simulink model "simuMotorFeedforward3"  (R2014a)
settings: Solver=ode45  StartTime=0.0  StopTime=3  MaxStep=0.0001  RelTol=1e-3
values from neighbouring files (symbols this model uses):
  contr = param    [parametres.m]
undefined symbols (not defined in the file or in its folder): param
settings Model: Creator=Etienne  LastModifiedBy=Etienne

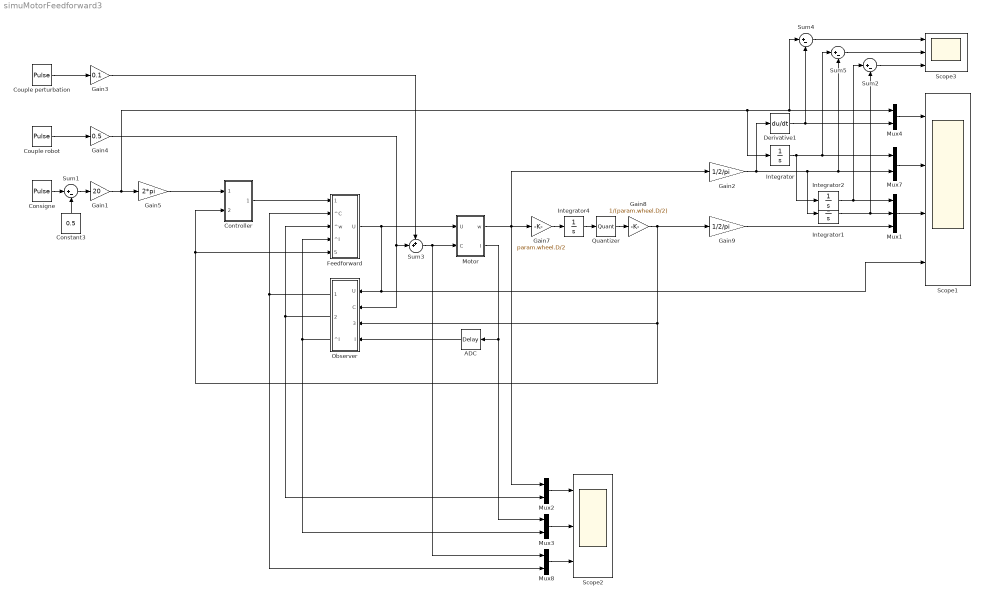
== system simuMotorFeedforward3 ==
  ADC : TransportDelay  DelayTime=param.adc.retard
  Consigne : DiscretePulseGenerator  PulseType=Time based  Period=1  PulseWidth=50  PhaseDelay=0.25/2
  Constant3 : Constant  Value=0.5
  Controller : Subsystem
  Couple perturbation : DiscretePulseGenerator  PulseType=Time based  Period=2/3  PulseWidth=50  PhaseDelay=0.3
  Couple robot : DiscretePulseGenerator  PulseType=Time based  Period=1.5  PulseWidth=50  PhaseDelay=0.1
  Derivative1 : Derivative
  Feedforward : Subsystem
  Gain1 : Gain  Gain=20
  Gain2 : Gain  Gain=1/2/pi
  Gain3 : Gain  Gain=0.1
  Gain4 : Gain  Gain=0.5
  Gain5 : Gain  Gain=2*pi
  Gain7 : Gain  Gain=param.wheel.D/2
  Gain8 : Gain  Gain=1/(param.wheel.D/2)
  Gain9 : Gain  Gain=1/2/pi
  Integrator{,1..2,4} (4 alike) : Integrator
  Motor : Subsystem
  Mux1 : Mux  Inputs=3
  Mux{2..4,7..8} (5 alike) : Mux  Inputs=2
  Observer : Subsystem
  Quantizer : Quantizer  QuantizationInterval=param.codeur.resolution
  Scope1 : Scope  NumInputPorts=4
      settings: TimeRange=3  YMin=-250~-2~-0.5~-30  YMax=200~4~4~30  SaveName=ScopeData2  MaxDataPoints=500000
  Scope2 : Scope  NumInputPorts=3
      settings: TimeRange=3  YMin=-10~-6~-1.5  YMax=25~10~3  MaxDataPoints=500000
  Scope3 : Scope  NumInputPorts=3
      settings: TimeRange=3  YMin=-100~-0.4~-0.005  YMax=150~0.3~0.004000000000000001  SaveName=ScopeData3  MaxDataPoints=500000
  Sum{1..2,4..5} (4 alike) : Sum  Inputs=|+-
  Sum3 : Sum  Inputs=++|
  wires:
  Couple perturbation/1 -> Gain3/1
  Motor/2(I) -> Mux3/1, ADC/1
  Consigne/1 -> Sum1/1
  Sum1/1 -> Gain1/1
  Constant3/1 -> Sum1/2
  Gain2/1 -> Derivative1/1, Integrator1/1, Sum5/2, Mux7/2
  Feedforward/1(U) -> Motor/1(U), Scope1/4, Observer/1(U)
  ADC/1 -> Observer/4(I)
  Mux4/1 -> Scope1/1
  Observer/2(^w) -> Mux2/2, Feedforward/3(^w)
  Observer/3(^I) -> Mux3/2, Feedforward/4(^I)
  Gain1/1 -> Gain5/1, Integrator/1, Mux4/1, Sum4/1
  Gain3/1 -> Sum3/1
  Derivative1/1 -> Mux4/2, Sum4/2
  Mux7/1 -> Scope1/2
  Integrator/1 -> Sum5/1, Mux7/1, Integrator2/1
  Sum4/1 -> Scope3/1
  Sum5/1 -> Scope3/2
  Mux1/1 -> Scope1/3
  Integrator1/1 -> Mux1/2, Sum2/2
  Integrator2/1 -> Mux1/1, Sum2/1
  Sum2/1 -> Scope3/3
  Gain4/1 -> Sum3/2, Observer/2(C)
  Integrator4/1 -> Quantizer/1
  Quantizer/1 -> Gain8/1
  Gain9/1 -> Mux1/3
  Motor/1(w) -> Gain7/1, Gain2/1, Mux2/1
  Gain7/1 -> Integrator4/1
  Mux2/1 -> Scope2/1
  Mux3/1 -> Scope2/2
  Mux8/1 -> Scope2/3
  Gain5/1 -> Controller/1(cons)
  Sum3/1 -> Motor/2(C), Mux8/1
  Couple robot/1 -> Gain4/1
  Controller/1(out) -> Feedforward/1(cons)
  Gain8/1 -> Feedforward/5(teta), Controller/2(teta), Observer/3(teta), Gain9/1
  Observer/1(^C) -> Feedforward/2(^C), Mux8/2

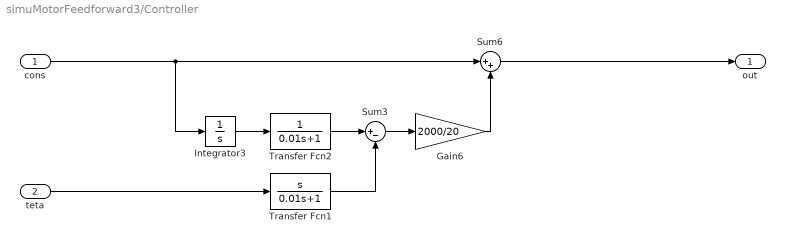
== system simuMotorFeedforward3/Controller ==
  cons : Inport
  teta : Inport  Port=2
  Gain6 : Gain  Gain=2000/20
  Integrator3 : Integrator
  Sum3 : Sum  Inputs=|+-
  Sum6 : Sum  Inputs=|++
  Transfer Fcn1 : TransferFcn  Numerator=[1 0]  Denominator=[0.01 1]
  Transfer Fcn2 : TransferFcn  Denominator=[0.01 1]
  out : Outport
  wires:
  Transfer Fcn2/1 -> Sum3/1
  teta/1 -> Transfer Fcn1/1
  Integrator3/1 -> Transfer Fcn2/1
  cons/1 -> Sum6/1, Integrator3/1
  Sum3/1 -> Gain6/1
  Sum6/1 -> out/1
  Gain6/1 -> Sum6/2
  Transfer Fcn1/1 -> Sum3/2

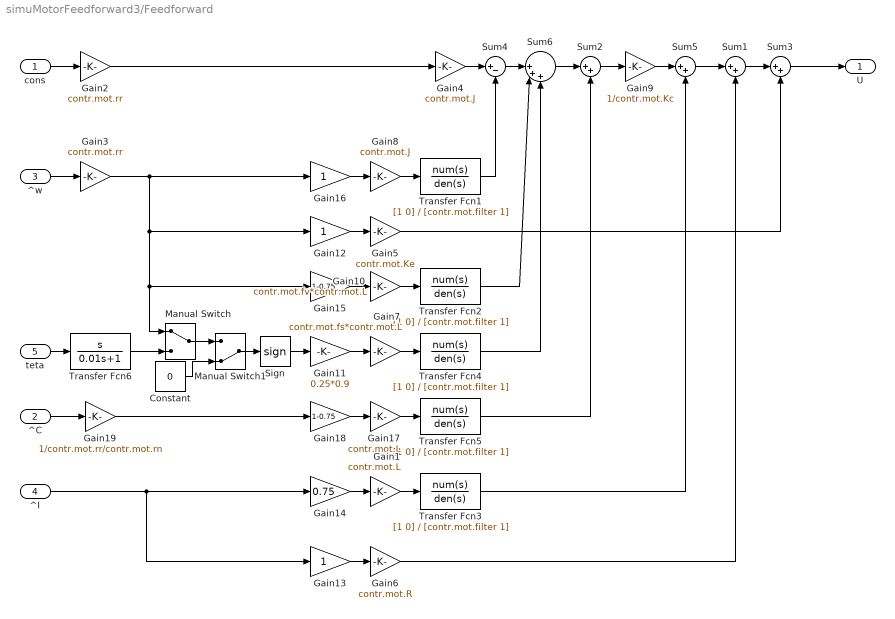
== system simuMotorFeedforward3/Feedforward ==
  cons : Inport
  ^C : Inport  Port=2
  ^w : Inport  Port=3
  ^I : Inport  Port=4
  teta : Inport  Port=5
  Constant : Constant  Value=0
  Gain1 : Gain  Gain=contr.mot.L
  Gain10 : Gain  Gain=contr.mot.fv*contr.mot.L
  Gain11 : Gain  Gain=0.25*0.9
  Gain12 : Gain
  Gain13 : Gain
  Gain14 : Gain  Gain=0.75
  Gain15 : Gain  Gain=1-0.75
  Gain16 : Gain
  Gain17 : Gain  Gain=contr.mot.L
  Gain18 : Gain  Gain=1-0.75
  Gain19 : Gain  Gain=1/contr.mot.rr/contr.mot.rn
  Gain2 : Gain  Gain=contr.mot.rr
  Gain3 : Gain  Gain=contr.mot.rr
  Gain4 : Gain  Gain=contr.mot.J
  Gain5 : Gain  Gain=contr.mot.Ke
  Gain6 : Gain  Gain=contr.mot.R
  Gain7 : Gain  Gain=contr.mot.fs*contr.mot.L
  Gain8 : Gain  Gain=contr.mot.J
  Gain9 : Gain  Gain=1/contr.mot.Kc
  Manual Switch : ManualSwitch
  Manual Switch1 : ManualSwitch  CurrentSetting=0
  Sign : Signum  ZeroCross=off
  Sum{1..3,5} (4 alike) : Sum  Inputs=|++
  Sum4 : Sum  Inputs=|+-
  Sum6 : Sum  Inputs=||+++
  Transfer Fcn{1..5} (5 alike) : TransferFcn  Numerator=[1 0]  Denominator=[contr.mot.filter 1]
  Transfer Fcn6 : TransferFcn  Numerator=[1 0]  Denominator=[0.01 1]
  U : Outport
  wires:
  Gain5/1 -> Sum3/2
  Gain8/1 -> Transfer Fcn1/1
  Gain2/1 -> Gain4/1
  Sum1/1 -> Sum3/1
  Gain6/1 -> Sum1/2
  Sum3/1 -> U/1
  Transfer Fcn1/1 -> Sum4/2
  Transfer Fcn3/1 -> Sum5/2
  Sum5/1 -> Sum1/1
  Gain12/1 -> Gain5/1
  Gain9/1 -> Sum5/1
  Gain1/1 -> Transfer Fcn3/1
  Gain15/1 -> Gain10/1
  Gain16/1 -> Gain8/1
  Gain13/1 -> Gain6/1
  Gain14/1 -> Gain1/1
  Sum4/1 -> Sum6/1
  cons/1 -> Gain2/1
  ^w/1 -> Gain3/1
  ^I/1 -> Gain14/1, Gain13/1
  Gain4/1 -> Sum4/1
  Gain10/1 -> Transfer Fcn2/1
  Transfer Fcn2/1 -> Sum6/2
  Gain7/1 -> Transfer Fcn4/1
  Gain11/1 -> Gain7/1
  Sign/1 -> Gain11/1
  Transfer Fcn4/1 -> Sum6/3
  Gain17/1 -> Transfer Fcn5/1
  Gain18/1 -> Gain17/1
  Sum6/1 -> Sum2/1
  Sum2/1 -> Gain9/1
  Transfer Fcn5/1 -> Sum2/2
  ^C/1 -> Gain19/1
  teta/1 -> Transfer Fcn6/1
  Gain19/1 -> Gain18/1
  Gain3/1 -> Gain16/1, Gain12/1, Gain15/1, Manual Switch/1
  Manual Switch/1 -> Manual Switch1/1
  Transfer Fcn6/1 -> Manual Switch/2
  Constant/1 -> Manual Switch1/2
  Manual Switch1/1 -> Sign/1

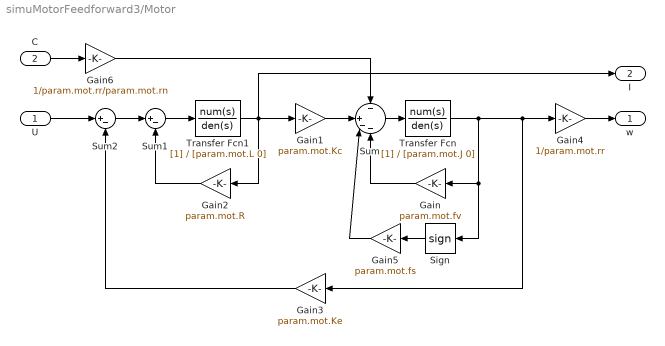
== system simuMotorFeedforward3/Motor ==
  U : Inport
  C : Inport  Port=2
  Gain : Gain  Gain=param.mot.fv
  Gain1 : Gain  Gain=param.mot.Kc
  Gain2 : Gain  Gain=param.mot.R
  Gain3 : Gain  Gain=param.mot.Ke
  Gain4 : Gain  Gain=1/param.mot.rr
  Gain5 : Gain  Gain=param.mot.fs
  Gain6 : Gain  Gain=1/param.mot.rr/param.mot.rn
  Sign : Signum  ZeroCross=off
  Sum : Sum  Inputs=-|+--
  Sum1 : Sum  Inputs=|+-
  Sum2 : Sum  Inputs=|+-
  Transfer Fcn : TransferFcn  Denominator=[param.mot.J 0]
  Transfer Fcn1 : TransferFcn  Denominator=[param.mot.L 0]
  w : Outport
  I : Outport  Port=2
  wires:
  Gain1/1 -> Sum/2
  Transfer Fcn/1 -> Gain3/1, Gain4/1, Sign/1, Gain/1
  Gain3/1 -> Sum2/2
  Sum2/1 -> Sum1/1
  Gain2/1 -> Sum1/2
  Sum1/1 -> Transfer Fcn1/1
  U/1 -> Sum2/1
  C/1 -> Gain6/1
  Gain6/1 -> Sum/1
  Gain4/1 -> w/1
  Sum/1 -> Transfer Fcn/1
  Transfer Fcn1/1 -> Gain1/1, I/1, Gain2/1
  Sign/1 -> Gain5/1
  Gain/1 -> Sum/4
  Gain5/1 -> Sum/3

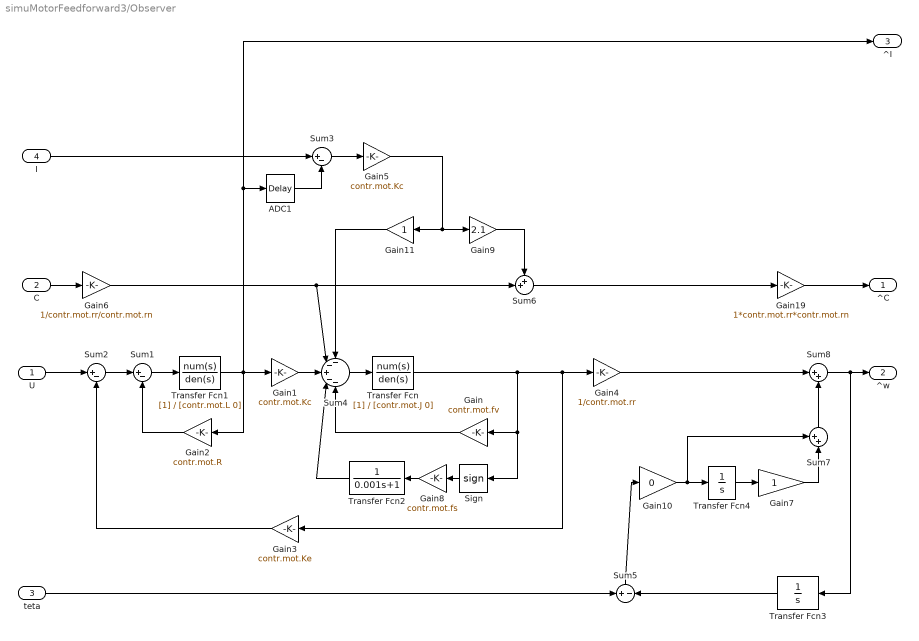
== system simuMotorFeedforward3/Observer ==
  U : Inport
  C : Inport  Port=2
  teta : Inport  Port=3
  I : Inport  Port=4
  ADC1 : TransportDelay  DelayTime=contr.adc.retard
  Gain : Gain  Gain=contr.mot.fv
  Gain1 : Gain  Gain=contr.mot.Kc
  Gain10 : Gain  Gain=0
  Gain11 : Gain
  Gain19 : Gain  Gain=1*contr.mot.rr*contr.mot.rn
  Gain2 : Gain  Gain=contr.mot.R
  Gain3 : Gain  Gain=contr.mot.Ke
  Gain4 : Gain  Gain=1/contr.mot.rr
  Gain5 : Gain  Gain=contr.mot.Kc
  Gain6 : Gain  Gain=1/contr.mot.rr/contr.mot.rn
  Gain7 : Gain
  Gain8 : Gain  Gain=contr.mot.fs
  Gain9 : Gain  Gain=2.1
  Sign : Signum  ZeroCross=off
  Sum1 : Sum  Inputs=|+-
  Sum2 : Sum  Inputs=|+-
  Sum3 : Sum  Inputs=|+-
  Sum4 : Sum  Inputs=--+--
  Sum5 : Sum  Inputs=+|-
  Sum6 : Sum  Inputs=++|
  Sum7 : Sum  Inputs=++|
  Sum8 : Sum  Inputs=|++
  Transfer Fcn : TransferFcn  Denominator=[contr.mot.J 0]
  Transfer Fcn1 : TransferFcn  Denominator=[contr.mot.L 0]
  Transfer Fcn2 : TransferFcn  Denominator=[0.001 1]
  Transfer Fcn3 : TransferFcn  Denominator=[1 0]
  Transfer Fcn4 : TransferFcn  Denominator=[1 0]
  ^C : Outport
  ^w : Outport  Port=2
  ^I : Outport  Port=3
  wires:
  Transfer Fcn/1 -> Gain3/1, Gain4/1, Gain/1, Sign/1
  Gain3/1 -> Sum2/2
  Sum2/1 -> Sum1/1
  Sum1/1 -> Transfer Fcn1/1
  U/1 -> Sum2/1
  C/1 -> Gain6/1
  Sum3/1 -> Gain5/1
  Gain2/1 -> Sum1/2
  Sign/1 -> Gain8/1
  Sum4/1 -> Transfer Fcn/1
  Gain8/1 -> Transfer Fcn2/1
  teta/1 -> Sum5/1
  Transfer Fcn3/1 -> Sum5/2
  Sum5/1 -> Gain10/1
  Gain4/1 -> Sum8/1
  Sum8/1 -> Transfer Fcn3/1, ^w/1
  Transfer Fcn4/1 -> Gain7/1
  Gain10/1 -> Sum7/1, Transfer Fcn4/1
  Gain6/1 -> Sum4/2, Sum6/2
  Gain7/1 -> Sum7/2
  Sum7/1 -> Sum8/2
  Sum6/1 -> Gain19/1
  I/1 -> Sum3/1
  ADC1/1 -> Sum3/2
  Gain19/1 -> ^C/1
  Transfer Fcn1/1 -> ^I/1, ADC1/1, Gain2/1, Gain1/1
  Gain/1 -> Sum4/5
  Gain1/1 -> Sum4/3
  Gain9/1 -> Sum6/1
  Gain5/1 -> Gain11/1, Gain9/1
  Gain11/1 -> Sum4/1
  Transfer Fcn2/1 -> Sum4/4
